simulink model "Simulink_Model"  (R2018a)
settings: Solver=VariableStepAuto  StartTime=0.0  StopTime=T_v(n+1)  MaxStep=0.001
values from neighbouring files (symbols this model uses):
  euler_v = deg2rad(euler_v)    [Simulation_Parameters.m]
  I_b = [151612935.5/10^9	       -12035.62/10^9        -9941.66/10^9 ... (first row only)    [Simulation_Parameters.m]
  I_new = I_sys - I_rw_z * (a1_R1_to_0*a1_0_to_R1+a2_R2_to_0*a2_0_to_R2+a3_R3_to_0*a3_0_to_R3)    [Simulation_Parameters.m]
  I_rw_z = 418129.72/10^9    (= 0.00041812972)    [Simulation_Parameters.m]
  I_single_rw = [220358.07/10^9         0               0 ... (first row only)    [Simulation_Parameters.m]
  I_st = [118601552.74/10^9	       -491524.85/10^9         95420.21/10^9 ... (first row only)    [Simulation_Parameters.m]
  I_sys = [177776253.6/10^9         -12078.47/10^9	        -9914.94/10^9 ... (first row only)    [Simulation_Parameters.m]
  Kd_r = [d;d;d]    [Simulation_Parameters.m]
  Kd_t = [d;d]    [Simulation_Parameters.m]
  Kp_r = [p;p;p]    [Simulation_Parameters.m]
  Kp_t = [p;p]    [Simulation_Parameters.m]
  m_b = 16.9927    [Simulation_Parameters.m]
  m_rw = 0.24806    [Simulation_Parameters.m]
  m_st = 9.48989    [Simulation_Parameters.m]
  m_tot = m_sys + m_st    (= 27.22678)    [Simulation_Parameters.m]
  mf = 1    [Simulation_Parameters.m]
  n = 4    [Simulation_Parameters.m]
  R_0_to_1 = [sqrt(2)/2 0.5 0.5; -sqrt(2)/2 0.5 0.5; 0 -sqrt(2)/2 sqrt(2)/2]    [Simulation_Parameters.m]
  R_1_to_0 = inv(R_0_to_1)    [Simulation_Parameters.m]
undefined symbols (not defined in the file or in its folder): k_phi_1, k_phi_2, k_phi_3, k_psi_1, k_psi_2, k_psi_3, k_theta_1, k_theta_2, k_theta_3, k_x_1, k_x_2, k_x_3, k_y_1, k_y_2, k_y_3, pos_v, t_acc, t_no_acc, t_t_acc, t_t_no_acc, T_v, X, Y, Z
libraries: nesl_utility x20, sm_lib x16, vrlib x2
(part 2 of 2)

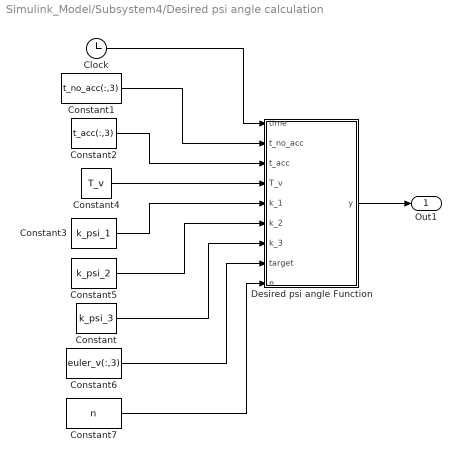
== system Simulink_Model/Subsystem4/Desired psi angle calculation ==
  Clock : Clock
  Constant : Constant  Value=k_psi_3
  Constant1 : Constant  Value=t_no_acc(:,3)
  Constant2 : Constant  Value=t_acc(:,3)
  Constant3 : Constant  Value=k_psi_1
  Constant4 : Constant  Value=T_v
  Constant5 : Constant  Value=k_psi_2
  Constant6 : Constant  Value=euler_v(:,3)
  Constant7 : Constant  Value=n
  Desired psi angle Function : MATLAB Function  TreatAsAtomicUnit=on
  Out1 : Outport
  wires:
  Constant1/1 -> Desired psi angle Function/2(t_no_acc)
  Constant5/1 -> Desired psi angle Function/6(k_2)
  Constant3/1 -> Desired psi angle Function/5(k_1)
  Constant2/1 -> Desired psi angle Function/3(t_acc)
  Desired psi angle Function/1(y) -> Out1/1
  Constant4/1 -> Desired psi angle Function/4(T_v)
  Constant/1 -> Desired psi angle Function/7(k_3)
  Clock/1 -> Desired psi angle Function/1(time)
  Constant7/1 -> Desired psi angle Function/9(n)
  Constant6/1 -> Desired psi angle Function/8(target)

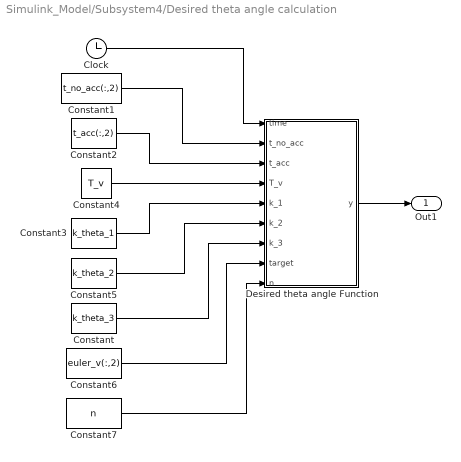
== system Simulink_Model/Subsystem4/Desired theta angle calculation ==
  Clock : Clock
  Constant : Constant  Value=k_theta_3
  Constant1 : Constant  Value=t_no_acc(:,2)
  Constant2 : Constant  Value=t_acc(:,2)
  Constant3 : Constant  Value=k_theta_1
  Constant4 : Constant  Value=T_v
  Constant5 : Constant  Value=k_theta_2
  Constant6 : Constant  Value=euler_v(:,2)
  Constant7 : Constant  Value=n
  Desired theta angle Function : MATLAB Function  TreatAsAtomicUnit=on
  Out1 : Outport
  wires:
  Constant1/1 -> Desired theta angle Function/2(t_no_acc)
  Constant5/1 -> Desired theta angle Function/6(k_2)
  Constant3/1 -> Desired theta angle Function/5(k_1)
  Constant2/1 -> Desired theta angle Function/3(t_acc)
  Desired theta angle Function/1(y) -> Out1/1
  Constant4/1 -> Desired theta angle Function/4(T_v)
  Constant/1 -> Desired theta angle Function/7(k_3)
  Clock/1 -> Desired theta angle Function/1(time)
  Constant7/1 -> Desired theta angle Function/9(n)
  Constant6/1 -> Desired theta angle Function/8(target)

== system Simulink_Model/Subsystem5/Desired x acceleration calculation ==
  Clock : Clock
  Constant : Constant  Value=k_x_3
  Constant1 : Constant  Value=t_t_no_acc(:,1)
  Constant2 : Constant  Value=t_t_acc(:,1)
  Constant3 : Constant  Value=k_x_1
  Constant4 : Constant  Value=T_v
  Constant5 : Constant  Value=k_x_2
  Constant6 : Constant  Value=pos_v(:,1)
  Constant7 : Constant  Value=n
  Desired x acceleration Function : MATLAB Function  TreatAsAtomicUnit=on
  Out1 : Outport
  wires:
  Clock/1 -> Desired x acceleration Function/1(time)
  Desired x acceleration Function/1(y) -> Out1/1
  Constant1/1 -> Desired x acceleration Function/2(t_no_acc)
  Constant2/1 -> Desired x acceleration Function/3(t_acc)
  Constant4/1 -> Desired x acceleration Function/4(T_v)
  Constant/1 -> Desired x acceleration Function/7(k_3)
  Constant5/1 -> Desired x acceleration Function/6(k_2)
  Constant3/1 -> Desired x acceleration Function/5(k_1)
  Constant6/1 -> Desired x acceleration Function/8(target)
  Constant7/1 -> Desired x acceleration Function/9(n)

== system Simulink_Model/Subsystem5/Desired y acceleration calculation ==
  Clock : Clock
  Constant : Constant  Value=k_y_3
  Constant1 : Constant  Value=t_t_no_acc(:,2)
  Constant2 : Constant  Value=t_t_acc(:,2)
  Constant3 : Constant  Value=k_y_1
  Constant4 : Constant  Value=T_v
  Constant5 : Constant  Value=k_y_2
  Constant6 : Constant  Value=pos_v(:,2)
  Constant7 : Constant  Value=n
  Desired y acceleration Function : MATLAB Function  TreatAsAtomicUnit=on
  Out1 : Outport
  wires:
  Constant5/1 -> Desired y acceleration Function/6(k_2)
  Constant4/1 -> Desired y acceleration Function/4(T_v)
  Constant1/1 -> Desired y acceleration Function/2(t_no_acc)
  Desired y acceleration Function/1(y) -> Out1/1
  Constant6/1 -> Desired y acceleration Function/8(target)
  Constant3/1 -> Desired y acceleration Function/5(k_1)
  Clock/1 -> Desired y acceleration Function/1(time)
  Constant2/1 -> Desired y acceleration Function/3(t_acc)
  Constant/1 -> Desired y acceleration Function/7(k_3)
  Constant7/1 -> Desired y acceleration Function/9(n)

== system Simulink_Model/Subsystem6/Desired phi angular acceleration calculation ==
  Clock : Clock
  Constant : Constant  Value=k_phi_3
  Constant1 : Constant  Value=t_no_acc(:,1)
  Constant2 : Constant  Value=t_acc(:,1)
  Constant3 : Constant  Value=k_phi_1
  Constant4 : Constant  Value=T_v
  Constant5 : Constant  Value=k_phi_2
  Constant6 : Constant  Value=euler_v(:,1)
  Constant7 : Constant  Value=n
  Desired phi angular acceleration Function : MATLAB Function  TreatAsAtomicUnit=on
  Out1 : Outport
  wires:
  Clock/1 -> Desired phi angular acceleration Function/1(time)
  Desired phi angular acceleration Function/1(y) -> Out1/1
  Constant1/1 -> Desired phi angular acceleration Function/2(t_no_acc)
  Constant2/1 -> Desired phi angular acceleration Function/3(t_acc)
  Constant4/1 -> Desired phi angular acceleration Function/4(T_v)
  Constant/1 -> Desired phi angular acceleration Function/7(k_3)
  Constant5/1 -> Desired phi angular acceleration Function/6(k_2)
  Constant3/1 -> Desired phi angular acceleration Function/5(k_1)
  Constant6/1 -> Desired phi angular acceleration Function/8(target)
  Constant7/1 -> Desired phi angular acceleration Function/9(n)

== system Simulink_Model/Subsystem6/Desired psi angular acceleration calculation ==
  Clock : Clock
  Constant : Constant  Value=k_psi_3
  Constant1 : Constant  Value=t_no_acc(:,3)
  Constant2 : Constant  Value=t_acc(:,3)
  Constant3 : Constant  Value=k_psi_1
  Constant4 : Constant  Value=T_v
  Constant5 : Constant  Value=k_psi_2
  Constant6 : Constant  Value=euler_v(:,3)
  Constant7 : Constant  Value=n
  Desired psi angular acceleration Function : MATLAB Function  TreatAsAtomicUnit=on
  Out1 : Outport
  wires:
  Constant1/1 -> Desired psi angular acceleration Function/2(t_no_acc)
  Constant5/1 -> Desired psi angular acceleration Function/6(k_2)
  Constant3/1 -> Desired psi angular acceleration Function/5(k_1)
  Constant2/1 -> Desired psi angular acceleration Function/3(t_acc)
  Desired psi angular acceleration Function/1(y) -> Out1/1
  Constant4/1 -> Desired psi angular acceleration Function/4(T_v)
  Constant/1 -> Desired psi angular acceleration Function/7(k_3)
  Clock/1 -> Desired psi angular acceleration Function/1(time)
  Constant7/1 -> Desired psi angular acceleration Function/9(n)
  Constant6/1 -> Desired psi angular acceleration Function/8(target)

== system Simulink_Model/Subsystem6/Desired theta angular acceleration calculation ==
  Clock : Clock
  Constant : Constant  Value=k_theta_3
  Constant1 : Constant  Value=t_no_acc(:,2)
  Constant2 : Constant  Value=t_acc(:,2)
  Constant3 : Constant  Value=k_theta_1
  Constant4 : Constant  Value=T_v
  Constant5 : Constant  Value=k_theta_2
  Constant6 : Constant  Value=euler_v(:,2)
  Constant7 : Constant  Value=n
  Desired theta angular acceleration Function : MATLAB Function  TreatAsAtomicUnit=on
  Out1 : Outport
  wires:
  Constant1/1 -> Desired theta angular acceleration Function/2(t_no_acc)
  Constant5/1 -> Desired theta angular acceleration Function/6(k_2)
  Constant3/1 -> Desired theta angular acceleration Function/5(k_1)
  Constant2/1 -> Desired theta angular acceleration Function/3(t_acc)
  Desired theta angular acceleration Function/1(y) -> Out1/1
  Constant4/1 -> Desired theta angular acceleration Function/4(T_v)
  Constant/1 -> Desired theta angular acceleration Function/7(k_3)
  Clock/1 -> Desired theta angular acceleration Function/1(time)
  Constant7/1 -> Desired theta angular acceleration Function/9(n)
  Constant6/1 -> Desired theta angular acceleration Function/8(target)

== matlab function Simulink_Model/R Matrix Calculation ==
  data: phi_a input; y output; theta_a input; psi_a input
function y = fcn(phi_a,theta_a,psi_a)

if cos(theta_a) == 0
    theta_a = theta_a + 0.0001;
end
 
 E_r = [            cos(theta_a)*cos(psi_a)                                      cos(theta_a)*sin(psi_a)                              -sin(theta_a);
        sin(phi_a)*sin(theta_a)*cos(psi_a)-cos(phi_a)*sin(psi_a)     sin(phi_a)*sin(theta_a)*sin(psi_a)+cos(phi_a)*cos(psi_a)     sin(phi_a)*cos(theta_a);
        cos(phi_a)*sin(theta_a)*cos(psi_a)+sin(phi_a)*sin(psi_a)     cos(phi_a)*sin(theta_a)*sin(psi_a)-sin(phi_a)*cos(psi_a)     cos(phi_a)*cos(theta_a)];
 
 

y = E_r;

== matlab function Simulink_Model/Inverse E Matrix Calculation/E^(-1) Matrix Calculation ==
  data: phi_a input; y output; theta_a input; psi_a input
function y = fcn(phi_a,theta_a,psi_a)

if cos(theta_a) == 0
    theta_a = theta_a + 0.0001;
end
 
 E_r = [1  tan(theta_a)*sin(phi_a)  cos(phi_a)*tan(theta_a);
        0         cos(phi_a)                -sin(phi_a);
        0  sin(phi_a)/cos(theta_a)  cos(phi_a)/cos(theta_a)];
 
 

y = E_r;

== matlab function Simulink_Model/Thruster Force Calculation/Thruster Analogue Force Calculator ==
  data: Ft output; t_open output; Fx input; Fy input; Fz input; Tx input; Ty input; Tz input; Forces output
function [Ft,t_open,Forces]= fcn(Fx,Fy,Fz,Tx,Ty,Tz)

f = [Fx;Fy;Fz;Tx;Ty;Tz];

d = 0.2335;
T = 0.1;

A = [-1  cosd(60)   cosd(60)  0        0            0;
      0  sind(60)  -sind(60)  0        0            0;
      0     0          0      1        1            1;
      0     0          0      d  -d*cosd(30)  -d*cosd(30);
      0     0          0      0  -d*sind(30)   d*sind(30);
      d     d          d      0        0            0   ];

Ft_d = inv(A)*f;

Ft = [0;0;0;0;0;0;0;0;0;0;0;0];
t_open = [0;0;0;0;0;0;0;0;0;0;0;0];

if Ft_d(1) == 0
    
    Ft(1) = 0;
    Ft(2) = 0;
    t_open(1) = 0;
    t_open(2) = 0;
    
elseif Ft_d(1) > 0
    
    Ft(1) = 1;
    Ft(2) = 0;
    t_open(1) = abs(Ft_d(1)*T);
    t_open(2) = 0;
    
else
    
    Ft(1) = 0;
    Ft(2) = 1;
    t_open(1) = 0;
    t_open(2) = abs(Ft_d(1)*T);
    
end

%%%%%%%%%%%%%%%%%%%%%%%%%%%%%%%%%%%%%%%%%%%%%%%%%%%%%%%%%%%%%%

if Ft_d(2) == 0
    
    Ft(3) = 0;
    Ft(4) = 0;
    t_open(3) = 0;
    t_open(4) = 0;
    
elseif Ft_d(2) > 0
    
    Ft(3) = 1;
    Ft(4) = 0;
    t_open(3) = abs(Ft_d(2)*T);
    t_open(4) = 0;
    
else
    
    Ft(3) = 0;
    Ft(4) = 1;
    t_open(3) = 0;
    t_open(4) = abs(Ft_d(2)*T);
    
end

%%%%%%%%%%%%%%%%%%%%%%%%%%%%%%%%%%%%%%%%%%%%%%%%%%%%%%%%%%%%%%

if Ft_d(3) == 0
    
    Ft(5) = 0;
    Ft(6) = 0;
    t_open(5) = 0;
    t_open(6) = 0;
    
elseif Ft_d(3) > 0
    
    Ft(5) = 1;
    Ft(6) = 0;
    t_open(5) = abs(Ft_d(3)*T);
    t_open(6) = 0;
    
else
    
    Ft(5) = 0;
    Ft(6) = 1;
    t_open(5) = 0;
    t_open(6) = abs(Ft_d(3)*T);
    
end

%%%%%%%%%%%%%%%%%%%%%%%%%%%%%%%%%%%%%%%%%%%%%%%%%%%%%%%%%%%%%%

if Ft_d(4) == 0
    
    Ft(7) = 0;
    Ft(8) = 0;
    t_open(7) = 0;
    t_open(8) = 0;
    
elseif Ft_d(4) > 0
    
    Ft(7) = 1;
    Ft(8) = 0;
    t_open(7) = abs(Ft_d(4)*T);
    t_open(8) = 0;
    
else
    
    Ft(7) = 0;
    Ft(8) = 1;
    t_open(7) = 0;
    t_open(8) = abs(Ft_d(4)*T);
    
end

%%%%%%%%%%%%%%%%%%%%%%%%%%%%%%%%%%%%%%%%%%%%%%%%%%%%%%%%%%%%%%

if Ft_d(5) == 0
    
    Ft(9) = 0;
    Ft(10) = 0;
    t_open(9) = 0;
    t_open(10) = 0;
    
elseif Ft_d(5) > 0
    
    Ft(9) = 1;
    Ft(10) = 0;
    t_open(9) = abs(Ft_d(5)*T);
    t_open(10) = 0;
    
else
    
    Ft(9) = 0;
    Ft(10) = 1;
    t_open(9) = 0;
    t_open(10) = abs(Ft_d(5)*T);
    
end

%%%%%%%%%%%%%%%%%%%%%%%%%%%%%%%%%%%%%%%%%%%%%%%%%%%%%%%%%%%%%%

if Ft_d(6) == 0
    
    Ft(11) = 0;
    Ft(12) = 0;
    t_open(11) = 0;
    t_open(12) = 0;
    
elseif Ft_d(6) > 0
    
    Ft(11) = 1;
    Ft(12) = 0;
    t_open(11) = abs(Ft_d(6)*T);
    t_open(12) = 0;
    
else
    
    Ft(11) = 0;
    Ft(12) = 1;
    t_open(11) = 0;
    t_open(12) = abs(Ft_d(6)*T);
    
end

for i = 1:6
    if Ft_d(i) > 1
        
        Ft_d(i) = 1;
        
    elseif Ft_d(i) < -1
        
        Ft_d(i) = -1;
        
    end
end

FT = A * Ft_d;

Forces = [FT(1);FT(2);FT(3);FT(4);FT(5);FT(6);0;0;0;0;0;0];

== matlab function Simulink_Model/Thruster Force Calculation/Thruster PWM Force Calculator ==
  data: time input; Ft input; Ftp output; t_open input
function Ftp = fcn(time,Ft,t_open)

P = 0.1;

t = time - fix(time/P)*P;
Ftp = [0;0;0;0;0;0;0;0;0;0;0;0];

for i = 1:12
    if t <= t_open(i)
        Ftp(i) = Ft(i);
    else
        Ftp(i) = 0;
    end
end

== matlab function Simulink_Model/Subsystem4/Desired theta angle calculation/Desired theta angle Function ==
  data: time input; t_no_acc input; t_acc input; T_v input; y output; k_1 input; k_2 input; k_3 input; target input; n input
function y = fcn(time,t_no_acc,t_acc,T_v,k_1,k_2,k_3,target,n)

j = 1;

for i = 1:n
    if time >= T_v(i)
        j = i;
    end
end


if time <= 0
    angle_d = 0;
    w_d = 0;
    a_d = 0;
elseif time <= T_v(j) + t_acc(j)
    angle_d =     k_1(j,1)*time^7 +    k_1(j,2)*time^6 +    k_1(j,3)*time^5 +    k_1(j,4)*time^4 +   k_1(j,5)*time^3 +   k_1(j,6)*time^2 + k_1(j,7)*time^1 + k_1(j,8);
        w_d =   7*k_1(j,1)*time^6 +  6*k_1(j,2)*time^5 +  5*k_1(j,3)*time^4 +  4*k_1(j,4)*time^3 + 3*k_1(j,5)*time^2 + 2*k_1(j,6)*time^1 + k_1(j,7);
        a_d =  42*k_1(j,1)*time^5 + 30*k_1(j,2)*time^4 + 20*k_1(j,3)*time^3 + 12*k_1(j,4)*time^2 + 6*k_1(j,5)*time^1 + 2*k_1(j,6);
elseif time <= T_v(j) + t_acc(j)+t_no_acc(j)
    angle_d =     k_2(j,1)*time^7 +    k_2(j,2)*time^6 +    k_2(j,3)*time^5 +    k_2(j,4)*time^4 +   k_2(j,5)*time^3 +   k_2(j,6)*time^2 + k_2(j,7)*time^1 + k_2(j,8);
        w_d =   7*k_2(j,1)*time^6 +  6*k_2(j,2)*time^5 +  5*k_2(j,3)*time^4 +  4*k_2(j,4)*time^3 + 3*k_2(j,5)*time^2 + 2*k_2(j,6)*time^1 + k_2(j,7);
        a_d =  42*k_2(j,1)*time^5 + 30*k_2(j,2)*time^4 + 20*k_2(j,3)*time^3 + 12*k_2(j,4)*time^2 + 6*k_2(j,5)*time^1 + 2*k_2(j,6);
elseif time <= T_v(j+1)
    angle_d =     k_3(j,1)*time^7 +    k_3(j,2)*time^6 +    k_3(j,3)*time^5 +    k_3(j,4)*time^4 +   k_3(j,5)*time^3 +   k_3(j,6)*time^2 + k_3(j,7)*time^1 + k_3(j,8);
        w_d =   7*k_3(j,1)*time^6 +  6*k_3(j,2)*time^5 +  5*k_3(j,3)*time^4 +  4*k_3(j,4)*time^3 + 3*k_3(j,5)*time^2 + 2*k_3(j,6)*time^1 + k_3(j,7);
        a_d =  42*k_3(j,1)*time^5 + 30*k_3(j,2)*time^4 + 20*k_3(j,3)*time^3 + 12*k_3(j,4)*time^2 + 6*k_3(j,5)*time^1 + 2*k_3(j,6);
else
    angle_d = target(j+1);
        w_d = 0;
        a_d = 0;
end

y = angle_d;

== matlab function Simulink_Model/Subsystem1/Desired x velocity calculation/Desired x velocity Function ==
  data: time input; t_no_acc input; t_acc input; T_v input; y output; k_1 input; k_2 input; k_3 input; target input; n input
function y = fcn(time,t_no_acc,t_acc,T_v,k_1,k_2,k_3,target,n)

j = 1;

for i = 1:n
    if time >= T_v(i)
        j = i;
    end
end


if time <= 0
    angle_d = 0;
    w_d = 0;
    a_d = 0;
elseif time <= T_v(j) + t_acc(j)
    angle_d =     k_1(j,1)*time^7 +    k_1(j,2)*time^6 +    k_1(j,3)*time^5 +    k_1(j,4)*time^4 +   k_1(j,5)*time^3 +   k_1(j,6)*time^2 + k_1(j,7)*time^1 + k_1(j,8);
        w_d =   7*k_1(j,1)*time^6 +  6*k_1(j,2)*time^5 +  5*k_1(j,3)*time^4 +  4*k_1(j,4)*time^3 + 3*k_1(j,5)*time^2 + 2*k_1(j,6)*time^1 + k_1(j,7);
        a_d =  42*k_1(j,1)*time^5 + 30*k_1(j,2)*time^4 + 20*k_1(j,3)*time^3 + 12*k_1(j,4)*time^2 + 6*k_1(j,5)*time^1 + 2*k_1(j,6);
elseif time <= T_v(j) + t_acc(j)+t_no_acc(j)
    angle_d =     k_2(j,1)*time^7 +    k_2(j,2)*time^6 +    k_2(j,3)*time^5 +    k_2(j,4)*time^4 +   k_2(j,5)*time^3 +   k_2(j,6)*time^2 + k_2(j,7)*time^1 + k_2(j,8);
        w_d =   7*k_2(j,1)*time^6 +  6*k_2(j,2)*time^5 +  5*k_2(j,3)*time^4 +  4*k_2(j,4)*time^3 + 3*k_2(j,5)*time^2 + 2*k_2(j,6)*time^1 + k_2(j,7);
        a_d =  42*k_2(j,1)*time^5 + 30*k_2(j,2)*time^4 + 20*k_2(j,3)*time^3 + 12*k_2(j,4)*time^2 + 6*k_2(j,5)*time^1 + 2*k_2(j,6);
elseif time <= T_v(j+1)
    angle_d =     k_3(j,1)*time^7 +    k_3(j,2)*time^6 +    k_3(j,3)*time^5 +    k_3(j,4)*time^4 +   k_3(j,5)*time^3 +   k_3(j,6)*time^2 + k_3(j,7)*time^1 + k_3(j,8);
        w_d =   7*k_3(j,1)*time^6 +  6*k_3(j,2)*time^5 +  5*k_3(j,3)*time^4 +  4*k_3(j,4)*time^3 + 3*k_3(j,5)*time^2 + 2*k_3(j,6)*time^1 + k_3(j,7);
        a_d =  42*k_3(j,1)*time^5 + 30*k_3(j,2)*time^4 + 20*k_3(j,3)*time^3 + 12*k_3(j,4)*time^2 + 6*k_3(j,5)*time^1 + 2*k_3(j,6);
else
    angle_d = target(j+1);
        w_d = 0;
        a_d = 0;
end

y = w_d;

== matlab function Simulink_Model/Subsystem1/Desired y velocity calculation/Desired y velocity Function ==
  data: time input; t_no_acc input; t_acc input; T_v input; y output; k_1 input; k_2 input; k_3 input; target input; n input
function y = fcn(time,t_no_acc,t_acc,T_v,k_1,k_2,k_3,target,n)

j = 1;

for i = 1:n
    if time >= T_v(i)
        j = i;
    end
end


if time <= 0
    angle_d = 0;
    w_d = 0;
    a_d = 0;
elseif time <= T_v(j) + t_acc(j)
    angle_d =     k_1(j,1)*time^7 +    k_1(j,2)*time^6 +    k_1(j,3)*time^5 +    k_1(j,4)*time^4 +   k_1(j,5)*time^3 +   k_1(j,6)*time^2 + k_1(j,7)*time^1 + k_1(j,8);
        w_d =   7*k_1(j,1)*time^6 +  6*k_1(j,2)*time^5 +  5*k_1(j,3)*time^4 +  4*k_1(j,4)*time^3 + 3*k_1(j,5)*time^2 + 2*k_1(j,6)*time^1 + k_1(j,7);
        a_d =  42*k_1(j,1)*time^5 + 30*k_1(j,2)*time^4 + 20*k_1(j,3)*time^3 + 12*k_1(j,4)*time^2 + 6*k_1(j,5)*time^1 + 2*k_1(j,6);
elseif time <= T_v(j) + t_acc(j)+t_no_acc(j)
    angle_d =     k_2(j,1)*time^7 +    k_2(j,2)*time^6 +    k_2(j,3)*time^5 +    k_2(j,4)*time^4 +   k_2(j,5)*time^3 +   k_2(j,6)*time^2 + k_2(j,7)*time^1 + k_2(j,8);
        w_d =   7*k_2(j,1)*time^6 +  6*k_2(j,2)*time^5 +  5*k_2(j,3)*time^4 +  4*k_2(j,4)*time^3 + 3*k_2(j,5)*time^2 + 2*k_2(j,6)*time^1 + k_2(j,7);
        a_d =  42*k_2(j,1)*time^5 + 30*k_2(j,2)*time^4 + 20*k_2(j,3)*time^3 + 12*k_2(j,4)*time^2 + 6*k_2(j,5)*time^1 + 2*k_2(j,6);
elseif time <= T_v(j+1)
    angle_d =     k_3(j,1)*time^7 +    k_3(j,2)*time^6 +    k_3(j,3)*time^5 +    k_3(j,4)*time^4 +   k_3(j,5)*time^3 +   k_3(j,6)*time^2 + k_3(j,7)*time^1 + k_3(j,8);
        w_d =   7*k_3(j,1)*time^6 +  6*k_3(j,2)*time^5 +  5*k_3(j,3)*time^4 +  4*k_3(j,4)*time^3 + 3*k_3(j,5)*time^2 + 2*k_3(j,6)*time^1 + k_3(j,7);
        a_d =  42*k_3(j,1)*time^5 + 30*k_3(j,2)*time^4 + 20*k_3(j,3)*time^3 + 12*k_3(j,4)*time^2 + 6*k_3(j,5)*time^1 + 2*k_3(j,6);
else
    angle_d = target(j+1);
        w_d = 0;
        a_d = 0;
end

y = w_d;

== matlab function Simulink_Model/Subsystem2/Desired y position calculation/Desired y position Function ==
  data: time input; t_no_acc input; t_acc input; T_v input; y output; k_1 input; k_2 input; k_3 input; target input; n input
function y = fcn(time,t_no_acc,t_acc,T_v,k_1,k_2,k_3,target,n)

j = 1;

for i = 1:n
    if time >= T_v(i)
        j = i;
    end
end


if time <= 0
    angle_d = 0;
    w_d = 0;
    a_d = 0;
elseif time <= T_v(j) + t_acc(j)
    angle_d =     k_1(j,1)*time^7 +    k_1(j,2)*time^6 +    k_1(j,3)*time^5 +    k_1(j,4)*time^4 +   k_1(j,5)*time^3 +   k_1(j,6)*time^2 + k_1(j,7)*time^1 + k_1(j,8);
        w_d =   7*k_1(j,1)*time^6 +  6*k_1(j,2)*time^5 +  5*k_1(j,3)*time^4 +  4*k_1(j,4)*time^3 + 3*k_1(j,5)*time^2 + 2*k_1(j,6)*time^1 + k_1(j,7);
        a_d =  42*k_1(j,1)*time^5 + 30*k_1(j,2)*time^4 + 20*k_1(j,3)*time^3 + 12*k_1(j,4)*time^2 + 6*k_1(j,5)*time^1 + 2*k_1(j,6);
elseif time <= T_v(j) + t_acc(j)+t_no_acc(j)
    angle_d =     k_2(j,1)*time^7 +    k_2(j,2)*time^6 +    k_2(j,3)*time^5 +    k_2(j,4)*time^4 +   k_2(j,5)*time^3 +   k_2(j,6)*time^2 + k_2(j,7)*time^1 + k_2(j,8);
        w_d =   7*k_2(j,1)*time^6 +  6*k_2(j,2)*time^5 +  5*k_2(j,3)*time^4 +  4*k_2(j,4)*time^3 + 3*k_2(j,5)*time^2 + 2*k_2(j,6)*time^1 + k_2(j,7);
        a_d =  42*k_2(j,1)*time^5 + 30*k_2(j,2)*time^4 + 20*k_2(j,3)*time^3 + 12*k_2(j,4)*time^2 + 6*k_2(j,5)*time^1 + 2*k_2(j,6);
elseif time <= T_v(j+1)
    angle_d =     k_3(j,1)*time^7 +    k_3(j,2)*time^6 +    k_3(j,3)*time^5 +    k_3(j,4)*time^4 +   k_3(j,5)*time^3 +   k_3(j,6)*time^2 + k_3(j,7)*time^1 + k_3(j,8);
        w_d =   7*k_3(j,1)*time^6 +  6*k_3(j,2)*time^5 +  5*k_3(j,3)*time^4 +  4*k_3(j,4)*time^3 + 3*k_3(j,5)*time^2 + 2*k_3(j,6)*time^1 + k_3(j,7);
        a_d =  42*k_3(j,1)*time^5 + 30*k_3(j,2)*time^4 + 20*k_3(j,3)*time^3 + 12*k_3(j,4)*time^2 + 6*k_3(j,5)*time^1 + 2*k_3(j,6);
else
    angle_d = target(j+1);
        w_d = 0;
        a_d = 0;
end

y = angle_d;

== matlab function Simulink_Model/Subsystem5/Desired x acceleration calculation/Desired x acceleration Function ==
  data: time input; t_no_acc input; t_acc input; T_v input; y output; k_1 input; k_2 input; k_3 input; target input; n input
function y = fcn(time,t_no_acc,t_acc,T_v,k_1,k_2,k_3,target,n)

j = 1;

for i = 1:n
    if time >= T_v(i)
        j = i;
    end
end


if time <= 0
    angle_d = 0;
    w_d = 0;
    a_d = 0;
elseif time <= T_v(j) + t_acc(j)
    angle_d =     k_1(j,1)*time^7 +    k_1(j,2)*time^6 +    k_1(j,3)*time^5 +    k_1(j,4)*time^4 +   k_1(j,5)*time^3 +   k_1(j,6)*time^2 + k_1(j,7)*time^1 + k_1(j,8);
        w_d =   7*k_1(j,1)*time^6 +  6*k_1(j,2)*time^5 +  5*k_1(j,3)*time^4 +  4*k_1(j,4)*time^3 + 3*k_1(j,5)*time^2 + 2*k_1(j,6)*time^1 + k_1(j,7);
        a_d =  42*k_1(j,1)*time^5 + 30*k_1(j,2)*time^4 + 20*k_1(j,3)*time^3 + 12*k_1(j,4)*time^2 + 6*k_1(j,5)*time^1 + 2*k_1(j,6);
elseif time <= T_v(j) + t_acc(j)+t_no_acc(j)
    angle_d =     k_2(j,1)*time^7 +    k_2(j,2)*time^6 +    k_2(j,3)*time^5 +    k_2(j,4)*time^4 +   k_2(j,5)*time^3 +   k_2(j,6)*time^2 + k_2(j,7)*time^1 + k_2(j,8);
        w_d =   7*k_2(j,1)*time^6 +  6*k_2(j,2)*time^5 +  5*k_2(j,3)*time^4 +  4*k_2(j,4)*time^3 + 3*k_2(j,5)*time^2 + 2*k_2(j,6)*time^1 + k_2(j,7);
        a_d =  42*k_2(j,1)*time^5 + 30*k_2(j,2)*time^4 + 20*k_2(j,3)*time^3 + 12*k_2(j,4)*time^2 + 6*k_2(j,5)*time^1 + 2*k_2(j,6);
elseif time <= T_v(j+1)
    angle_d =     k_3(j,1)*time^7 +    k_3(j,2)*time^6 +    k_3(j,3)*time^5 +    k_3(j,4)*time^4 +   k_3(j,5)*time^3 +   k_3(j,6)*time^2 + k_3(j,7)*time^1 + k_3(j,8);
        w_d =   7*k_3(j,1)*time^6 +  6*k_3(j,2)*time^5 +  5*k_3(j,3)*time^4 +  4*k_3(j,4)*time^3 + 3*k_3(j,5)*time^2 + 2*k_3(j,6)*time^1 + k_3(j,7);
        a_d =  42*k_3(j,1)*time^5 + 30*k_3(j,2)*time^4 + 20*k_3(j,3)*time^3 + 12*k_3(j,4)*time^2 + 6*k_3(j,5)*time^1 + 2*k_3(j,6);
else
    angle_d = target(j+1);
        w_d = 0;
        a_d = 0;
end

y = a_d;

== matlab function Simulink_Model/Subsystem5/Desired y acceleration calculation/Desired y acceleration Function ==
  data: time input; t_no_acc input; t_acc input; T_v input; y output; k_1 input; k_2 input; k_3 input; target input; n input
function y = fcn(time,t_no_acc,t_acc,T_v,k_1,k_2,k_3,target,n)

j = 1;

for i = 1:n
    if time >= T_v(i)
        j = i;
    end
end


if time <= 0
    angle_d = 0;
    w_d = 0;
    a_d = 0;
elseif time <= T_v(j) + t_acc(j)
    angle_d =     k_1(j,1)*time^7 +    k_1(j,2)*time^6 +    k_1(j,3)*time^5 +    k_1(j,4)*time^4 +   k_1(j,5)*time^3 +   k_1(j,6)*time^2 + k_1(j,7)*time^1 + k_1(j,8);
        w_d =   7*k_1(j,1)*time^6 +  6*k_1(j,2)*time^5 +  5*k_1(j,3)*time^4 +  4*k_1(j,4)*time^3 + 3*k_1(j,5)*time^2 + 2*k_1(j,6)*time^1 + k_1(j,7);
        a_d =  42*k_1(j,1)*time^5 + 30*k_1(j,2)*time^4 + 20*k_1(j,3)*time^3 + 12*k_1(j,4)*time^2 + 6*k_1(j,5)*time^1 + 2*k_1(j,6);
elseif time <= T_v(j) + t_acc(j)+t_no_acc(j)
    angle_d =     k_2(j,1)*time^7 +    k_2(j,2)*time^6 +    k_2(j,3)*time^5 +    k_2(j,4)*time^4 +   k_2(j,5)*time^3 +   k_2(j,6)*time^2 + k_2(j,7)*time^1 + k_2(j,8);
        w_d =   7*k_2(j,1)*time^6 +  6*k_2(j,2)*time^5 +  5*k_2(j,3)*time^4 +  4*k_2(j,4)*time^3 + 3*k_2(j,5)*time^2 + 2*k_2(j,6)*time^1 + k_2(j,7);
        a_d =  42*k_2(j,1)*time^5 + 30*k_2(j,2)*time^4 + 20*k_2(j,3)*time^3 + 12*k_2(j,4)*time^2 + 6*k_2(j,5)*time^1 + 2*k_2(j,6);
elseif time <= T_v(j+1)
    angle_d =     k_3(j,1)*time^7 +    k_3(j,2)*time^6 +    k_3(j,3)*time^5 +    k_3(j,4)*time^4 +   k_3(j,5)*time^3 +   k_3(j,6)*time^2 + k_3(j,7)*time^1 + k_3(j,8);
        w_d =   7*k_3(j,1)*time^6 +  6*k_3(j,2)*time^5 +  5*k_3(j,3)*time^4 +  4*k_3(j,4)*time^3 + 3*k_3(j,5)*time^2 + 2*k_3(j,6)*time^1 + k_3(j,7);
        a_d =  42*k_3(j,1)*time^5 + 30*k_3(j,2)*time^4 + 20*k_3(j,3)*time^3 + 12*k_3(j,4)*time^2 + 6*k_3(j,5)*time^1 + 2*k_3(j,6);
else
    angle_d = target(j+1);
        w_d = 0;
        a_d = 0;
end

y = a_d;

== matlab function Simulink_Model/Subsystem3/Desired phi angular velocity calculation/Desired phi angular velocity Function ==
  data: time input; t_no_acc input; t_acc input; T_v input; y output; k_1 input; k_2 input; k_3 input; target input; n input
function y = fcn(time,t_no_acc,t_acc,T_v,k_1,k_2,k_3,target,n)

j = 1;

for i = 1:n
    if time >= T_v(i)
        j = i;
    end
end


if time <= 0
    angle_d = 0;
    w_d = 0;
    a_d = 0;
elseif time <= T_v(j) + t_acc(j)
    angle_d =     k_1(j,1)*time^7 +    k_1(j,2)*time^6 +    k_1(j,3)*time^5 +    k_1(j,4)*time^4 +   k_1(j,5)*time^3 +   k_1(j,6)*time^2 + k_1(j,7)*time^1 + k_1(j,8);
        w_d =   7*k_1(j,1)*time^6 +  6*k_1(j,2)*time^5 +  5*k_1(j,3)*time^4 +  4*k_1(j,4)*time^3 + 3*k_1(j,5)*time^2 + 2*k_1(j,6)*time^1 + k_1(j,7);
        a_d =  42*k_1(j,1)*time^5 + 30*k_1(j,2)*time^4 + 20*k_1(j,3)*time^3 + 12*k_1(j,4)*time^2 + 6*k_1(j,5)*time^1 + 2*k_1(j,6);
elseif time <= T_v(j) + t_acc(j)+t_no_acc(j)
    angle_d =     k_2(j,1)*time^7 +    k_2(j,2)*time^6 +    k_2(j,3)*time^5 +    k_2(j,4)*time^4 +   k_2(j,5)*time^3 +   k_2(j,6)*time^2 + k_2(j,7)*time^1 + k_2(j,8);
        w_d =   7*k_2(j,1)*time^6 +  6*k_2(j,2)*time^5 +  5*k_2(j,3)*time^4 +  4*k_2(j,4)*time^3 + 3*k_2(j,5)*time^2 + 2*k_2(j,6)*time^1 + k_2(j,7);
        a_d =  42*k_2(j,1)*time^5 + 30*k_2(j,2)*time^4 + 20*k_2(j,3)*time^3 + 12*k_2(j,4)*time^2 + 6*k_2(j,5)*time^1 + 2*k_2(j,6);
elseif time <= T_v(j+1)
    angle_d =     k_3(j,1)*time^7 +    k_3(j,2)*time^6 +    k_3(j,3)*time^5 +    k_3(j,4)*time^4 +   k_3(j,5)*time^3 +   k_3(j,6)*time^2 + k_3(j,7)*time^1 + k_3(j,8);
        w_d =   7*k_3(j,1)*time^6 +  6*k_3(j,2)*time^5 +  5*k_3(j,3)*time^4 +  4*k_3(j,4)*time^3 + 3*k_3(j,5)*time^2 + 2*k_3(j,6)*time^1 + k_3(j,7);
        a_d =  42*k_3(j,1)*time^5 + 30*k_3(j,2)*time^4 + 20*k_3(j,3)*time^3 + 12*k_3(j,4)*time^2 + 6*k_3(j,5)*time^1 + 2*k_3(j,6);
else
    angle_d = target(j+1);
        w_d = 0;
        a_d = 0;
end

y = w_d;

== matlab function Simulink_Model/Subsystem3/Desired psi angular velocity calculation/Desired psi angular velocity Function ==
  data: time input; t_no_acc input; t_acc input; T_v input; y output; k_1 input; k_2 input; k_3 input; target input; n input
function y = fcn(time,t_no_acc,t_acc,T_v,k_1,k_2,k_3,target,n)

j = 1;

for i = 1:n
    if time >= T_v(i)
        j = i;
    end
end


if time <= 0
    angle_d = 0;
    w_d = 0;
    a_d = 0;
elseif time <= T_v(j) + t_acc(j)
    angle_d =     k_1(j,1)*time^7 +    k_1(j,2)*time^6 +    k_1(j,3)*time^5 +    k_1(j,4)*time^4 +   k_1(j,5)*time^3 +   k_1(j,6)*time^2 + k_1(j,7)*time^1 + k_1(j,8);
        w_d =   7*k_1(j,1)*time^6 +  6*k_1(j,2)*time^5 +  5*k_1(j,3)*time^4 +  4*k_1(j,4)*time^3 + 3*k_1(j,5)*time^2 + 2*k_1(j,6)*time^1 + k_1(j,7);
        a_d =  42*k_1(j,1)*time^5 + 30*k_1(j,2)*time^4 + 20*k_1(j,3)*time^3 + 12*k_1(j,4)*time^2 + 6*k_1(j,5)*time^1 + 2*k_1(j,6);
elseif time <= T_v(j) + t_acc(j)+t_no_acc(j)
    angle_d =     k_2(j,1)*time^7 +    k_2(j,2)*time^6 +    k_2(j,3)*time^5 +    k_2(j,4)*time^4 +   k_2(j,5)*time^3 +   k_2(j,6)*time^2 + k_2(j,7)*time^1 + k_2(j,8);
        w_d =   7*k_2(j,1)*time^6 +  6*k_2(j,2)*time^5 +  5*k_2(j,3)*time^4 +  4*k_2(j,4)*time^3 + 3*k_2(j,5)*time^2 + 2*k_2(j,6)*time^1 + k_2(j,7);
        a_d =  42*k_2(j,1)*time^5 + 30*k_2(j,2)*time^4 + 20*k_2(j,3)*time^3 + 12*k_2(j,4)*time^2 + 6*k_2(j,5)*time^1 + 2*k_2(j,6);
elseif time <= T_v(j+1)
    angle_d =     k_3(j,1)*time^7 +    k_3(j,2)*time^6 +    k_3(j,3)*time^5 +    k_3(j,4)*time^4 +   k_3(j,5)*time^3 +   k_3(j,6)*time^2 + k_3(j,7)*time^1 + k_3(j,8);
        w_d =   7*k_3(j,1)*time^6 +  6*k_3(j,2)*time^5 +  5*k_3(j,3)*time^4 +  4*k_3(j,4)*time^3 + 3*k_3(j,5)*time^2 + 2*k_3(j,6)*time^1 + k_3(j,7);
        a_d =  42*k_3(j,1)*time^5 + 30*k_3(j,2)*time^4 + 20*k_3(j,3)*time^3 + 12*k_3(j,4)*time^2 + 6*k_3(j,5)*time^1 + 2*k_3(j,6);
else
    angle_d = target(j+1);
        w_d = 0;
        a_d = 0;
end

y = w_d;

== matlab function Simulink_Model/Subsystem3/Desired theta angular velocity calculation/Desired theta angular velocity Function ==
  data: time input; t_no_acc input; t_acc input; T_v input; y output; k_1 input; k_2 input; k_3 input; target input; n input
function y = fcn(time,t_no_acc,t_acc,T_v,k_1,k_2,k_3,target,n)

j = 1;

for i = 1:n
    if time >= T_v(i)
        j = i;
    end
end


if time <= 0
    angle_d = 0;
    w_d = 0;
    a_d = 0;
elseif time <= T_v(j) + t_acc(j)
    angle_d =     k_1(j,1)*time^7 +    k_1(j,2)*time^6 +    k_1(j,3)*time^5 +    k_1(j,4)*time^4 +   k_1(j,5)*time^3 +   k_1(j,6)*time^2 + k_1(j,7)*time^1 + k_1(j,8);
        w_d =   7*k_1(j,1)*time^6 +  6*k_1(j,2)*time^5 +  5*k_1(j,3)*time^4 +  4*k_1(j,4)*time^3 + 3*k_1(j,5)*time^2 + 2*k_1(j,6)*time^1 + k_1(j,7);
        a_d =  42*k_1(j,1)*time^5 + 30*k_1(j,2)*time^4 + 20*k_1(j,3)*time^3 + 12*k_1(j,4)*time^2 + 6*k_1(j,5)*time^1 + 2*k_1(j,6);
elseif time <= T_v(j) + t_acc(j)+t_no_acc(j)
    angle_d =     k_2(j,1)*time^7 +    k_2(j,2)*time^6 +    k_2(j,3)*time^5 +    k_2(j,4)*time^4 +   k_2(j,5)*time^3 +   k_2(j,6)*time^2 + k_2(j,7)*time^1 + k_2(j,8);
        w_d =   7*k_2(j,1)*time^6 +  6*k_2(j,2)*time^5 +  5*k_2(j,3)*time^4 +  4*k_2(j,4)*time^3 + 3*k_2(j,5)*time^2 + 2*k_2(j,6)*time^1 + k_2(j,7);
        a_d =  42*k_2(j,1)*time^5 + 30*k_2(j,2)*time^4 + 20*k_2(j,3)*time^3 + 12*k_2(j,4)*time^2 + 6*k_2(j,5)*time^1 + 2*k_2(j,6);
elseif time <= T_v(j+1)
    angle_d =     k_3(j,1)*time^7 +    k_3(j,2)*time^6 +    k_3(j,3)*time^5 +    k_3(j,4)*time^4 +   k_3(j,5)*time^3 +   k_3(j,6)*time^2 + k_3(j,7)*time^1 + k_3(j,8);
        w_d =   7*k_3(j,1)*time^6 +  6*k_3(j,2)*time^5 +  5*k_3(j,3)*time^4 +  4*k_3(j,4)*time^3 + 3*k_3(j,5)*time^2 + 2*k_3(j,6)*time^1 + k_3(j,7);
        a_d =  42*k_3(j,1)*time^5 + 30*k_3(j,2)*time^4 + 20*k_3(j,3)*time^3 + 12*k_3(j,4)*time^2 + 6*k_3(j,5)*time^1 + 2*k_3(j,6);
else
    angle_d = target(j+1);
        w_d = 0;
        a_d = 0;
end

y = w_d;

== matlab function Simulink_Model/Subsystem4/Desired phi angle calculation/Desired phi angle Function ==
  data: time input; t_no_acc input; t_acc input; T_v input; y output; k_1 input; k_2 input; k_3 input; target input; n input
function y = fcn(time,t_no_acc,t_acc,T_v,k_1,k_2,k_3,target,n)

j = 1;

for i = 1:n
    if time >= T_v(i)
        j = i;
    end
end


if time <= 0
    angle_d = 0;
    w_d = 0;
    a_d = 0;
elseif time <= T_v(j) + t_acc(j)
    angle_d =     k_1(j,1)*time^7 +    k_1(j,2)*time^6 +    k_1(j,3)*time^5 +    k_1(j,4)*time^4 +   k_1(j,5)*time^3 +   k_1(j,6)*time^2 + k_1(j,7)*time^1 + k_1(j,8);
        w_d =   7*k_1(j,1)*time^6 +  6*k_1(j,2)*time^5 +  5*k_1(j,3)*time^4 +  4*k_1(j,4)*time^3 + 3*k_1(j,5)*time^2 + 2*k_1(j,6)*time^1 + k_1(j,7);
        a_d =  42*k_1(j,1)*time^5 + 30*k_1(j,2)*time^4 + 20*k_1(j,3)*time^3 + 12*k_1(j,4)*time^2 + 6*k_1(j,5)*time^1 + 2*k_1(j,6);
elseif time <= T_v(j) + t_acc(j)+t_no_acc(j)
    angle_d =     k_2(j,1)*time^7 +    k_2(j,2)*time^6 +    k_2(j,3)*time^5 +    k_2(j,4)*time^4 +   k_2(j,5)*time^3 +   k_2(j,6)*time^2 + k_2(j,7)*time^1 + k_2(j,8);
        w_d =   7*k_2(j,1)*time^6 +  6*k_2(j,2)*time^5 +  5*k_2(j,3)*time^4 +  4*k_2(j,4)*time^3 + 3*k_2(j,5)*time^2 + 2*k_2(j,6)*time^1 + k_2(j,7);
        a_d =  42*k_2(j,1)*time^5 + 30*k_2(j,2)*time^4 + 20*k_2(j,3)*time^3 + 12*k_2(j,4)*time^2 + 6*k_2(j,5)*time^1 + 2*k_2(j,6);
elseif time <= T_v(j+1)
    angle_d =     k_3(j,1)*time^7 +    k_3(j,2)*time^6 +    k_3(j,3)*time^5 +    k_3(j,4)*time^4 +   k_3(j,5)*time^3 +   k_3(j,6)*time^2 + k_3(j,7)*time^1 + k_3(j,8);
        w_d =   7*k_3(j,1)*time^6 +  6*k_3(j,2)*time^5 +  5*k_3(j,3)*time^4 +  4*k_3(j,4)*time^3 + 3*k_3(j,5)*time^2 + 2*k_3(j,6)*time^1 + k_3(j,7);
        a_d =  42*k_3(j,1)*time^5 + 30*k_3(j,2)*time^4 + 20*k_3(j,3)*time^3 + 12*k_3(j,4)*time^2 + 6*k_3(j,5)*time^1 + 2*k_3(j,6);
else
    angle_d = target(j+1);
        w_d = 0;
        a_d = 0;
end

y = angle_d;

== matlab function Simulink_Model/Subsystem4/Desired psi angle calculation/Desired psi angle Function ==
  data: time input; t_no_acc input; t_acc input; T_v input; y output; k_1 input; k_2 input; k_3 input; target input; n input
function y = fcn(time,t_no_acc,t_acc,T_v,k_1,k_2,k_3,target,n)

j = 1;

for i = 1:n
    if time >= T_v(i)
        j = i;
    end
end


if time <= 0
    angle_d = 0;
    w_d = 0;
    a_d = 0;
elseif time <= T_v(j) + t_acc(j)
    angle_d =     k_1(j,1)*time^7 +    k_1(j,2)*time^6 +    k_1(j,3)*time^5 +    k_1(j,4)*time^4 +   k_1(j,5)*time^3 +   k_1(j,6)*time^2 + k_1(j,7)*time^1 + k_1(j,8);
        w_d =   7*k_1(j,1)*time^6 +  6*k_1(j,2)*time^5 +  5*k_1(j,3)*time^4 +  4*k_1(j,4)*time^3 + 3*k_1(j,5)*time^2 + 2*k_1(j,6)*time^1 + k_1(j,7);
        a_d =  42*k_1(j,1)*time^5 + 30*k_1(j,2)*time^4 + 20*k_1(j,3)*time^3 + 12*k_1(j,4)*time^2 + 6*k_1(j,5)*time^1 + 2*k_1(j,6);
elseif time <= T_v(j) + t_acc(j)+t_no_acc(j)
    angle_d =     k_2(j,1)*time^7 +    k_2(j,2)*time^6 +    k_2(j,3)*time^5 +    k_2(j,4)*time^4 +   k_2(j,5)*time^3 +   k_2(j,6)*time^2 + k_2(j,7)*time^1 + k_2(j,8);
        w_d =   7*k_2(j,1)*time^6 +  6*k_2(j,2)*time^5 +  5*k_2(j,3)*time^4 +  4*k_2(j,4)*time^3 + 3*k_2(j,5)*time^2 + 2*k_2(j,6)*time^1 + k_2(j,7);
        a_d =  42*k_2(j,1)*time^5 + 30*k_2(j,2)*time^4 + 20*k_2(j,3)*time^3 + 12*k_2(j,4)*time^2 + 6*k_2(j,5)*time^1 + 2*k_2(j,6);
elseif time <= T_v(j+1)
    angle_d =     k_3(j,1)*time^7 +    k_3(j,2)*time^6 +    k_3(j,3)*time^5 +    k_3(j,4)*time^4 +   k_3(j,5)*time^3 +   k_3(j,6)*time^2 + k_3(j,7)*time^1 + k_3(j,8);
        w_d =   7*k_3(j,1)*time^6 +  6*k_3(j,2)*time^5 +  5*k_3(j,3)*time^4 +  4*k_3(j,4)*time^3 + 3*k_3(j,5)*time^2 + 2*k_3(j,6)*time^1 + k_3(j,7);
        a_d =  42*k_3(j,1)*time^5 + 30*k_3(j,2)*time^4 + 20*k_3(j,3)*time^3 + 12*k_3(j,4)*time^2 + 6*k_3(j,5)*time^1 + 2*k_3(j,6);
else
    angle_d = target(j+1);
        w_d = 0;
        a_d = 0;
end

y = angle_d;

== matlab function Simulink_Model/Subsystem6/Desired phi angular acceleration calculation/Desired phi angular acceleration Function ==
  data: time input; t_no_acc input; t_acc input; T_v input; y output; k_1 input; k_2 input; k_3 input; target input; n input
function y = fcn(time,t_no_acc,t_acc,T_v,k_1,k_2,k_3,target,n)

j = 1;

for i = 1:n
    if time >= T_v(i)
        j = i;
    end
end


if time <= 0
    angle_d = 0;
    w_d = 0;
    a_d = 0;
elseif time <= T_v(j) + t_acc(j)
    angle_d =     k_1(j,1)*time^7 +    k_1(j,2)*time^6 +    k_1(j,3)*time^5 +    k_1(j,4)*time^4 +   k_1(j,5)*time^3 +   k_1(j,6)*time^2 + k_1(j,7)*time^1 + k_1(j,8);
        w_d =   7*k_1(j,1)*time^6 +  6*k_1(j,2)*time^5 +  5*k_1(j,3)*time^4 +  4*k_1(j,4)*time^3 + 3*k_1(j,5)*time^2 + 2*k_1(j,6)*time^1 + k_1(j,7);
        a_d =  42*k_1(j,1)*time^5 + 30*k_1(j,2)*time^4 + 20*k_1(j,3)*time^3 + 12*k_1(j,4)*time^2 + 6*k_1(j,5)*time^1 + 2*k_1(j,6);
elseif time <= T_v(j) + t_acc(j)+t_no_acc(j)
    angle_d =     k_2(j,1)*time^7 +    k_2(j,2)*time^6 +    k_2(j,3)*time^5 +    k_2(j,4)*time^4 +   k_2(j,5)*time^3 +   k_2(j,6)*time^2 + k_2(j,7)*time^1 + k_2(j,8);
        w_d =   7*k_2(j,1)*time^6 +  6*k_2(j,2)*time^5 +  5*k_2(j,3)*time^4 +  4*k_2(j,4)*time^3 + 3*k_2(j,5)*time^2 + 2*k_2(j,6)*time^1 + k_2(j,7);
        a_d =  42*k_2(j,1)*time^5 + 30*k_2(j,2)*time^4 + 20*k_2(j,3)*time^3 + 12*k_2(j,4)*time^2 + 6*k_2(j,5)*time^1 + 2*k_2(j,6);
elseif time <= T_v(j+1)
    angle_d =     k_3(j,1)*time^7 +    k_3(j,2)*time^6 +    k_3(j,3)*time^5 +    k_3(j,4)*time^4 +   k_3(j,5)*time^3 +   k_3(j,6)*time^2 + k_3(j,7)*time^1 + k_3(j,8);
        w_d =   7*k_3(j,1)*time^6 +  6*k_3(j,2)*time^5 +  5*k_3(j,3)*time^4 +  4*k_3(j,4)*time^3 + 3*k_3(j,5)*time^2 + 2*k_3(j,6)*time^1 + k_3(j,7);
        a_d =  42*k_3(j,1)*time^5 + 30*k_3(j,2)*time^4 + 20*k_3(j,3)*time^3 + 12*k_3(j,4)*time^2 + 6*k_3(j,5)*time^1 + 2*k_3(j,6);
else
    angle_d = target(j+1);
        w_d = 0;
        a_d = 0;
end

y = a_d;

== matlab function Simulink_Model/MATLAB Function ==
  data: T_th_1 input; T_tr_1 output; T_th_2 input; T_th_3 input; w_1 input; w_2 input; w_3 input; T_tr_2 output; T_tr_3 output
function [T_tr_1,T_tr_2,T_tr_3] = fcn(T_th_1,T_th_2,T_th_3,w_1,w_2,w_3)

T_max = 0.0911;
T_max_1 = T_max;
T_max_2 = T_max;
T_max_3 = T_max;
T_max_c = T_max;

if (abs(w_1) * abs(T_th_1)) >= 50
    T_max_1 = 50/abs(w_1);
end

w_1 = w_1 * 60 / (2*pi);

if abs(w_1) >= 10000
    T_max_2 = 0;
end

if (abs(w_1)/265 + abs(T_th_1)*6920/265) >= 29.6
    T_max_3 = 265*29.6/6920 - abs(w_1)/6920;
end

if T_max_c > T_max_1
    T_max_c = T_max_1;
end
if T_max_c > T_max_2
    T_max_c = T_max_2;
end
if T_max_c > T_max_3
    T_max_c = T_max_3;
end

test_1 = T_max_c;

if abs(T_th_1) > T_max_c
    if T_th_1 >= 0
        T_tr_1 = T_max_c;
    else
        T_tr_1 = -T_max_c;
    end
else
    T_tr_1 = T_th_1;
end

%%%%%%%%%%%%%%%%%%%%%%%%%%%%%%%%%%%%%%%%%%%%%%%%%%%%%%%%%%%%%%%%%%%%

T_max_1 = T_max;
T_max_2 = T_max;
T_max_3 = T_max;
T_max_c = T_max;

if (abs(w_2) * abs(T_th_2)) >= 50
    T_max_1 = 50/abs(w_2);
end

w_2 = w_2 * 60 / (2*pi);

if abs(w_2) >= 10000
    T_max_2 = 0;
end

if (abs(w_2)/265 + abs(T_th_2)*6920/265) >= 24
    T_max_3 = 265*24/6920 - abs(w_2)/6920;
end

if T_max_c > T_max_1
    T_max_c = T_max_1;
end
if T_max_c > T_max_2
    T_max_c = T_max_2;
end
if T_max_c > T_max_3
    T_max_c = T_max_3;
end

test_2 = T_max_c;

if abs(T_th_2) > T_max_c
    if T_th_2 >= 0
        T_tr_2 = T_max_c;
    else
        T_tr_2 = -T_max_c;
    end
else
    T_tr_2 = T_th_2;
end

%%%%%%%%%%%%%%%%%%%%%%%%%%%%%%%%%%%%%%%%%%%%%%%%%%%%%%%%%%%%%%%%%%%%

T_max_1 = T_max;
T_max_2 = T_max;
T_max_3 = T_max;
T_max_c = T_max;

if (abs(w_3) * abs(T_th_3)) >= 50
    T_max_1 = 50/abs(w_3);
end

w_3 = w_3 * 60 / (2*pi);

if abs(w_3) >= 10000
    T_max_2 = 0;
end

if (abs(w_3)/265 + abs(T_th_3)*6920/265) >= 24
    T_max_3 = 265*24/6920 - abs(w_3)/6920;
end

if T_max_c > T_max_1
    T_max_c = T_max_1;
end
if T_max_c > T_max_2
    T_max_c = T_max_2;
end
if T_max_c > T_max_3
    T_max_c = T_max_3;
end

test_3 = T_max_c;

if abs(T_th_3) > T_max_c
    if T_th_3 >= 0
        T_tr_3 = T_max_c;
    else
        T_tr_3 = -T_max_c;
    end
else
    T_tr_3 = T_th_3;
end

== matlab function Simulink_Model/Internal Angle Calculation ==
  data: fc input; angle output
function angle = fcn(fc)

fxy = sqrt(fc(1)^2+fc(2)^2);
theta = atand(abs(fxy/(fc(3)+17.7369*9.81)));

angle = theta;

== matlab function Simulink_Model/Subsystem6/Desired psi angular acceleration calculation/Desired psi angular acceleration Function ==
  data: time input; t_no_acc input; t_acc input; T_v input; y output; k_1 input; k_2 input; k_3 input; target input; n input
function y = fcn(time,t_no_acc,t_acc,T_v,k_1,k_2,k_3,target,n)

j = 1;

for i = 1:n
    if time >= T_v(i)
        j = i;
    end
end


if time <= 0
    angle_d = 0;
    w_d = 0;
    a_d = 0;
elseif time <= T_v(j) + t_acc(j)
    angle_d =     k_1(j,1)*time^7 +    k_1(j,2)*time^6 +    k_1(j,3)*time^5 +    k_1(j,4)*time^4 +   k_1(j,5)*time^3 +   k_1(j,6)*time^2 + k_1(j,7)*time^1 + k_1(j,8);
        w_d =   7*k_1(j,1)*time^6 +  6*k_1(j,2)*time^5 +  5*k_1(j,3)*time^4 +  4*k_1(j,4)*time^3 + 3*k_1(j,5)*time^2 + 2*k_1(j,6)*time^1 + k_1(j,7);
        a_d =  42*k_1(j,1)*time^5 + 30*k_1(j,2)*time^4 + 20*k_1(j,3)*time^3 + 12*k_1(j,4)*time^2 + 6*k_1(j,5)*time^1 + 2*k_1(j,6);
elseif time <= T_v(j) + t_acc(j)+t_no_acc(j)
    angle_d =     k_2(j,1)*time^7 +    k_2(j,2)*time^6 +    k_2(j,3)*time^5 +    k_2(j,4)*time^4 +   k_2(j,5)*time^3 +   k_2(j,6)*time^2 + k_2(j,7)*time^1 + k_2(j,8);
        w_d =   7*k_2(j,1)*time^6 +  6*k_2(j,2)*time^5 +  5*k_2(j,3)*time^4 +  4*k_2(j,4)*time^3 + 3*k_2(j,5)*time^2 + 2*k_2(j,6)*time^1 + k_2(j,7);
        a_d =  42*k_2(j,1)*time^5 + 30*k_2(j,2)*time^4 + 20*k_2(j,3)*time^3 + 12*k_2(j,4)*time^2 + 6*k_2(j,5)*time^1 + 2*k_2(j,6);
elseif time <= T_v(j+1)
    angle_d =     k_3(j,1)*time^7 +    k_3(j,2)*time^6 +    k_3(j,3)*time^5 +    k_3(j,4)*time^4 +   k_3(j,5)*time^3 +   k_3(j,6)*time^2 + k_3(j,7)*time^1 + k_3(j,8);
        w_d =   7*k_3(j,1)*time^6 +  6*k_3(j,2)*time^5 +  5*k_3(j,3)*time^4 +  4*k_3(j,4)*time^3 + 3*k_3(j,5)*time^2 + 2*k_3(j,6)*time^1 + k_3(j,7);
        a_d =  42*k_3(j,1)*time^5 + 30*k_3(j,2)*time^4 + 20*k_3(j,3)*time^3 + 12*k_3(j,4)*time^2 + 6*k_3(j,5)*time^1 + 2*k_3(j,6);
else
    angle_d = target(j+1);
        w_d = 0;
        a_d = 0;
end

y = a_d;

== matlab function Simulink_Model/Subsystem6/Desired theta angular acceleration calculation/Desired theta angular acceleration Function ==
  data: time input; t_no_acc input; t_acc input; T_v input; y output; k_1 input; k_2 input; k_3 input; target input; n input
function y = fcn(time,t_no_acc,t_acc,T_v,k_1,k_2,k_3,target,n)

j = 1;

for i = 1:n
    if time >= T_v(i)
        j = i;
    end
end


if time <= 0
    angle_d = 0;
    w_d = 0;
    a_d = 0;
elseif time <= T_v(j) + t_acc(j)
    angle_d =     k_1(j,1)*time^7 +    k_1(j,2)*time^6 +    k_1(j,3)*time^5 +    k_1(j,4)*time^4 +   k_1(j,5)*time^3 +   k_1(j,6)*time^2 + k_1(j,7)*time^1 + k_1(j,8);
        w_d =   7*k_1(j,1)*time^6 +  6*k_1(j,2)*time^5 +  5*k_1(j,3)*time^4 +  4*k_1(j,4)*time^3 + 3*k_1(j,5)*time^2 + 2*k_1(j,6)*time^1 + k_1(j,7);
        a_d =  42*k_1(j,1)*time^5 + 30*k_1(j,2)*time^4 + 20*k_1(j,3)*time^3 + 12*k_1(j,4)*time^2 + 6*k_1(j,5)*time^1 + 2*k_1(j,6);
elseif time <= T_v(j) + t_acc(j)+t_no_acc(j)
    angle_d =     k_2(j,1)*time^7 +    k_2(j,2)*time^6 +    k_2(j,3)*time^5 +    k_2(j,4)*time^4 +   k_2(j,5)*time^3 +   k_2(j,6)*time^2 + k_2(j,7)*time^1 + k_2(j,8);
        w_d =   7*k_2(j,1)*time^6 +  6*k_2(j,2)*time^5 +  5*k_2(j,3)*time^4 +  4*k_2(j,4)*time^3 + 3*k_2(j,5)*time^2 + 2*k_2(j,6)*time^1 + k_2(j,7);
        a_d =  42*k_2(j,1)*time^5 + 30*k_2(j,2)*time^4 + 20*k_2(j,3)*time^3 + 12*k_2(j,4)*time^2 + 6*k_2(j,5)*time^1 + 2*k_2(j,6);
elseif time <= T_v(j+1)
    angle_d =     k_3(j,1)*time^7 +    k_3(j,2)*time^6 +    k_3(j,3)*time^5 +    k_3(j,4)*time^4 +   k_3(j,5)*time^3 +   k_3(j,6)*time^2 + k_3(j,7)*time^1 + k_3(j,8);
        w_d =   7*k_3(j,1)*time^6 +  6*k_3(j,2)*time^5 +  5*k_3(j,3)*time^4 +  4*k_3(j,4)*time^3 + 3*k_3(j,5)*time^2 + 2*k_3(j,6)*time^1 + k_3(j,7);
        a_d =  42*k_3(j,1)*time^5 + 30*k_3(j,2)*time^4 + 20*k_3(j,3)*time^3 + 12*k_3(j,4)*time^2 + 6*k_3(j,5)*time^1 + 2*k_3(j,6);
else
    angle_d = target(j+1);
        w_d = 0;
        a_d = 0;
end

y = a_d;

== matlab function Simulink_Model/Subsystem2/Desired x position calculation/Desired x position Function ==
  data: time input; t_no_acc input; t_acc input; T_v input; y output; k_1 input; k_2 input; k_3 input; target input; n input
function y = fcn(time,t_no_acc,t_acc,T_v,k_1,k_2,k_3,target,n)

j = 1;

for i = 1:n
    if time >= T_v(i)
        j = i;
    end
end


if time <= 0
    angle_d = 0;
    w_d = 0;
    a_d = 0;
elseif time <= T_v(j) + t_acc(j)
    angle_d =     k_1(j,1)*time^7 +    k_1(j,2)*time^6 +    k_1(j,3)*time^5 +    k_1(j,4)*time^4 +   k_1(j,5)*time^3 +   k_1(j,6)*time^2 + k_1(j,7)*time^1 + k_1(j,8);
        w_d =   7*k_1(j,1)*time^6 +  6*k_1(j,2)*time^5 +  5*k_1(j,3)*time^4 +  4*k_1(j,4)*time^3 + 3*k_1(j,5)*time^2 + 2*k_1(j,6)*time^1 + k_1(j,7);
        a_d =  42*k_1(j,1)*time^5 + 30*k_1(j,2)*time^4 + 20*k_1(j,3)*time^3 + 12*k_1(j,4)*time^2 + 6*k_1(j,5)*time^1 + 2*k_1(j,6);
elseif time <= T_v(j) + t_acc(j)+t_no_acc(j)
    angle_d =     k_2(j,1)*time^7 +    k_2(j,2)*time^6 +    k_2(j,3)*time^5 +    k_2(j,4)*time^4 +   k_2(j,5)*time^3 +   k_2(j,6)*time^2 + k_2(j,7)*time^1 + k_2(j,8);
        w_d =   7*k_2(j,1)*time^6 +  6*k_2(j,2)*time^5 +  5*k_2(j,3)*time^4 +  4*k_2(j,4)*time^3 + 3*k_2(j,5)*time^2 + 2*k_2(j,6)*time^1 + k_2(j,7);
        a_d =  42*k_2(j,1)*time^5 + 30*k_2(j,2)*time^4 + 20*k_2(j,3)*time^3 + 12*k_2(j,4)*time^2 + 6*k_2(j,5)*time^1 + 2*k_2(j,6);
elseif time <= T_v(j+1)
    angle_d =     k_3(j,1)*time^7 +    k_3(j,2)*time^6 +    k_3(j,3)*time^5 +    k_3(j,4)*time^4 +   k_3(j,5)*time^3 +   k_3(j,6)*time^2 + k_3(j,7)*time^1 + k_3(j,8);
        w_d =   7*k_3(j,1)*time^6 +  6*k_3(j,2)*time^5 +  5*k_3(j,3)*time^4 +  4*k_3(j,4)*time^3 + 3*k_3(j,5)*time^2 + 2*k_3(j,6)*time^1 + k_3(j,7);
        a_d =  42*k_3(j,1)*time^5 + 30*k_3(j,2)*time^4 + 20*k_3(j,3)*time^3 + 12*k_3(j,4)*time^2 + 6*k_3(j,5)*time^1 + 2*k_3(j,6);
else
    angle_d = target(j+1);
        w_d = 0;
        a_d = 0;
end

y = angle_d;
